simulink model "Układ_Obiekt_Ragulator_Obserwator"  (R2022b)
settings: Solver=VariableStepAuto  StartTime=0.0  StopTime=10.0  RelTol=1e-3
values from neighbouring files (symbols this model uses):
  K = acker(A, B, [s_b s_b s_b])    [Projekt_1.m]
  L = acker(A', C', [s_o s_o s_o])'    [Projekt_1.m]
  X_0 = [1; -5; 1]    [Projekt_1.m]
settings Model: Creator=pioro  LastModifiedBy=pioro

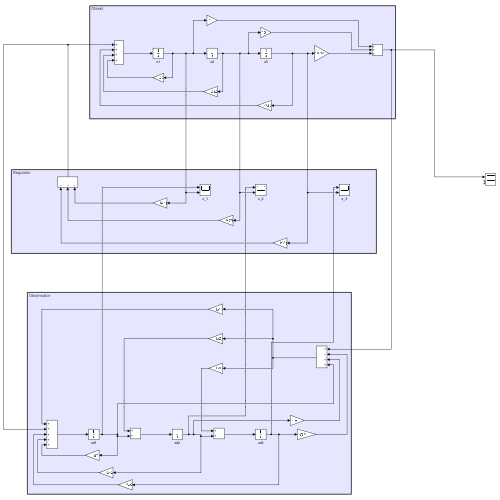
[thumbnail: Simulink's stored preview of the top-level diagram]
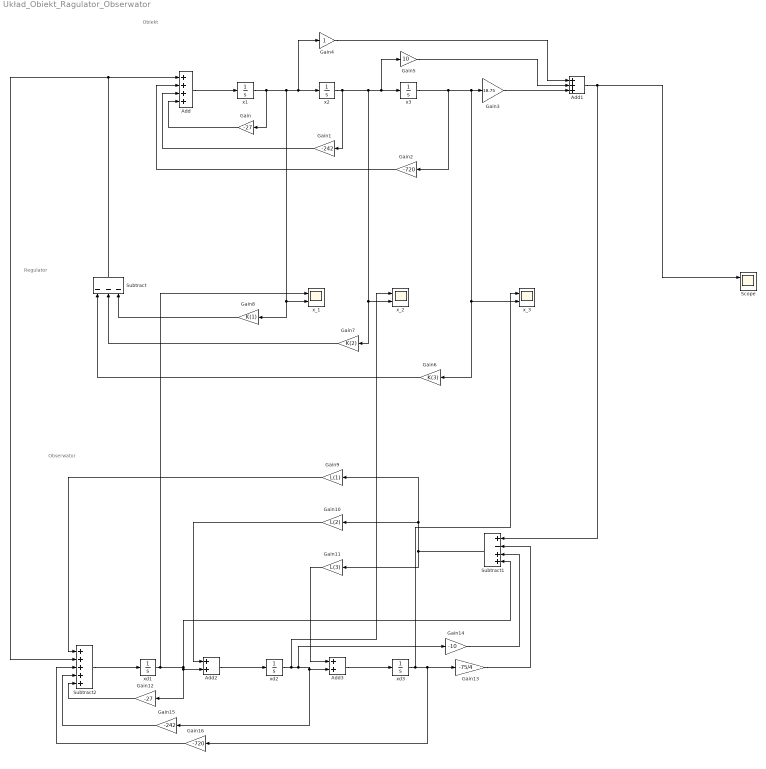
== system Układ_Obiekt_Ragulator_Obserwator ==
  note: Obserwator
  note: Regulator
  note: Obiekt
  Add : Sum  Inputs=++++
  Add1 : Sum  Inputs=+++
  Add2 : Sum
  Add3 : Sum
  Gain : Gain  Gain=-27
  Gain1 : Gain  Gain=-242
  Gain10 : Gain  Gain=L(2)
  Gain11 : Gain  Gain=L(3)
  Gain12 : Gain  Gain=-27
  Gain13 : Gain  Gain=-75/4
  Gain14 : Gain  Gain=-10
  Gain15 : Gain  Gain=-242
  Gain16 : Gain  Gain=-720
  Gain2 : Gain  Gain=-720
  Gain3 : Gain  Gain=18.75
  Gain4 : Gain
  Gain5 : Gain  Gain=10
  Gain6 : Gain  Gain=K(3)
  Gain7 : Gain  Gain=K(2)
  Gain8 : Gain  Gain=K(1)
  Gain9 : Gain  Gain=L(1)
  Scope : Scope  NumInputPorts=2
  Subtract : Sum  Inputs=---
  Subtract1 : Sum  Inputs=+-++
  Subtract2 : Sum  Inputs=+++++
  x1 : Integrator  InitialCondition=X_0(1)
  x2 : Integrator  InitialCondition=X_0(2)
  x3 : Integrator  InitialCondition=X_0(3)
  x_1 : Scope  NumInputPorts=2
  x_2 : Scope  NumInputPorts=2
  x_3 : Scope  NumInputPorts=2
  xd1 : Integrator
  xd2 : Integrator
  xd3 : Integrator
  wires:
  Gain3/1 -> Add1/3
  Gain5/1 -> Add1/2
  Gain4/1 -> Add1/1
  Gain/1 -> Add/4
  Add/1 -> x1/1
  Gain2/1 -> Add/2
  Gain1/1 -> Add/3
  Gain8/1 -> Subtract/3
  x2/1 -> x_2/2, Gain7/1, Gain5/1, x3/1, Gain1/1
  Gain6/1 -> Subtract/1
  Gain7/1 -> Subtract/2
  x1/1 -> Gain/1, x2/1, Gain4/1, x_1/2, Gain8/1
  x3/1 -> x_3/2, Gain6/1, Gain3/1, Gain2/1
  Add2/1 -> xd2/1
  Subtract2/1 -> xd1/1
  Gain9/1 -> Subtract2/1
  Gain15/1 -> Subtract2/4
  Add1/1 -> Subtract1/1, Scope/1
  Add3/1 -> xd3/1
  Gain12/1 -> Subtract2/5
  Gain16/1 -> Subtract2/3
  Gain10/1 -> Add2/1
  xd1/1 -> Gain12/1, Add2/2, Subtract1/4, x_1/1
  Subtract/1 -> Subtract2/2, Add/1
  Gain11/1 -> Add3/1
  Gain13/1 -> Subtract1/2
  Gain14/1 -> Subtract1/3
  xd2/1 -> Add3/2, Gain15/1, Gain14/1, x_2/1
  Subtract1/1 -> Gain9/1, Gain10/1, Gain11/1
  xd3/1 -> x_3/1, Gain16/1, Gain13/1
